simulink model "Feeder_1"  (Simulink 8.8)
settings: Solver=ode4  StartTime=0.0  StopTime=inf  FixedStep=Ts  RelTol=1e-3  EnableMultiTasking=on
PreLoadFcn:
  | Ts=125e-6;Core_Num = 0; np=1; nq=1; Vmin=.9;
PostLoadFcn:
  | Ts=125e-6;Core_Num = 0; np=1; nq=1; Vmin=.9;
InitFcn:
  | Ts=125e-6;Core_Num = 0; np=1; nq=1; Vmin=.9;
undefined symbols (not defined in the file or in its folder): another_event_name, DiscIntNeverNeededParam, I, j, Left, my_event_name, Right, type, V, X
libraries: powerlib x316, powerlib_meascontrol x227, simulink_extras x78, simulink x25, rtio_generic_c37_118 x22, ssn_lib x9, rtlab x6, powerlib_extras x3, artemis x1, rtio_opalrt_ml605ex1 x1, rtio_spectracom x1, rtio_generic_ethernet x1
(part 9 of 14)

== system Feeder_1/SM_NG/Single-Phase Dynamic Load41/model/Break  Alg. Loop1 ==
  In : Inport
  Complex to Real-Imag : ComplexToRealImag
  Real-Imag to Complex : RealImagToComplex
  imag : simulink_extras/Additional Linear/Transfer Fcn (with initial outputs)  N=[1]  D="[100e-6  1]"  Y0=imag(I1_init*exp(-j*Pha_V0*pi/180))  U0=imag(I1_init*exp(-j*Pha_V0*pi/180))
  real : simulink_extras/Additional Linear/Transfer Fcn (with initial outputs)  N=[1]  D="[100e-6  1]"  Y0=real(I1_init*exp(-j*Pha_V0*pi/180))  U0=real(I1_init*exp(-j*Pha_V0*pi/180))
  Out : Outport
  wires:
  Complex to Real-Imag/2 -> imag/1
  Complex to Real-Imag/1 -> real/1
  Real-Imag to Complex/1 -> Out/1
  In/1 -> Complex to Real-Imag/1
  imag/1 -> Real-Imag to Complex/2
  real/1 -> Real-Imag to Complex/1

== system Feeder_1/SM_NG/Single-Phase Dynamic Load41/model/PLL ==
  v (pu) : Inport
  freq (pu) : Inport  Port=2
  Gain : Gain  Gain=2*pi
  Gain1 : Gain  Gain=500
  Gain2 : Gain  Gain=freq
  IC : InitialCondition
  Integrator : Integrator
  Integrator1 : Integrator
  Product : Product  Inputs=**  RndMeth=Zero
  Sum1 : Sum  SaturateOnIntegerOverflow=on  InputSameDT=on  OutDataTypeStr=Inherit: Same as first input
  Trigonometric Function : Trigonometry  Operator=cos
  adaptive filter : Subsystem
  adaptive mean : Subsystem
  alpha (rad) : Outport
  wt : Outport  Port=2
  wires:
  freq (pu)/1 -> Gain2/1
  Gain2/1 -> adaptive filter/2(freq (Hz)), adaptive mean/2(freq (Hz)), Gain/1
  Trigonometric Function/1 -> Product/2
  adaptive mean/1(y) -> alpha (rad)/1
  Integrator1/1 -> Gain1/1
  Gain1/1 -> Sum1/1, adaptive mean/1(u)
  Sum1/1 -> Trigonometric Function/1
  Integrator/1 -> Sum1/2, wt/1
  Gain/1 -> Integrator/1
  adaptive filter/1(y) -> Integrator1/1
  Product/1 -> adaptive filter/1(u)
  v (pu)/1 -> IC/1
  IC/1 -> Product/1

== system Feeder_1/SM_NG/Single-Phase Dynamic Load41/model/Positive Sequence  current ==
  note: I1= (S/V1)'
  V1(pu) : Inport
  S_ext : Inport  Port=2
  Conj1 : Math  Operator=conj  SaturateOnIntegerOverflow=on
  Product : Product  Inputs=/*  SaturateOnIntegerOverflow=on  InputSameDT=on  OutDataTypeStr=Inherit: Same as first input
  pu>V : Gain  Gain=Vnom/sqrt(2)  SaturateOnIntegerOverflow=on  OutDataTypeStr=Inherit: Same as input  ParamDataTypeStr=Inherit: Same as input
  I1(A) : Outport
  wires:
  V1(pu)/1 -> pu>V/1
  Product/1 -> Conj1/1
  Conj1/1 -> I1(A)/1
  S_ext/1 -> Product/2
  pu>V/1 -> Product/1

== system Feeder_1/SM_NG/Single-Phase Dynamic Load42/model/Break  Alg. Loop1 ==
  In : Inport
  Complex to Real-Imag : ComplexToRealImag
  Real-Imag to Complex : RealImagToComplex
  imag : simulink_extras/Additional Linear/Transfer Fcn (with initial outputs)  N=[1]  D="[100e-6  1]"  Y0=imag(I1_init*exp(-j*Pha_V0*pi/180))  U0=imag(I1_init*exp(-j*Pha_V0*pi/180))
  real : simulink_extras/Additional Linear/Transfer Fcn (with initial outputs)  N=[1]  D="[100e-6  1]"  Y0=real(I1_init*exp(-j*Pha_V0*pi/180))  U0=real(I1_init*exp(-j*Pha_V0*pi/180))
  Out : Outport
  wires:
  Complex to Real-Imag/2 -> imag/1
  Complex to Real-Imag/1 -> real/1
  Real-Imag to Complex/1 -> Out/1
  In/1 -> Complex to Real-Imag/1
  imag/1 -> Real-Imag to Complex/2
  real/1 -> Real-Imag to Complex/1

== system Feeder_1/SM_NG/Single-Phase Dynamic Load42/model/PLL ==
  v (pu) : Inport
  freq (pu) : Inport  Port=2
  Gain : Gain  Gain=2*pi
  Gain1 : Gain  Gain=500
  Gain2 : Gain  Gain=freq
  IC : InitialCondition
  Integrator : Integrator
  Integrator1 : Integrator
  Product : Product  Inputs=**  RndMeth=Zero
  Sum1 : Sum  SaturateOnIntegerOverflow=on  InputSameDT=on  OutDataTypeStr=Inherit: Same as first input
  Trigonometric Function : Trigonometry  Operator=cos
  adaptive filter : Subsystem
  adaptive mean : Subsystem
  alpha (rad) : Outport
  wt : Outport  Port=2
  wires:
  freq (pu)/1 -> Gain2/1
  Gain2/1 -> adaptive filter/2(freq (Hz)), adaptive mean/2(freq (Hz)), Gain/1
  Trigonometric Function/1 -> Product/2
  adaptive mean/1(y) -> alpha (rad)/1
  Integrator1/1 -> Gain1/1
  Gain1/1 -> Sum1/1, adaptive mean/1(u)
  Sum1/1 -> Trigonometric Function/1
  Integrator/1 -> Sum1/2, wt/1
  Gain/1 -> Integrator/1
  adaptive filter/1(y) -> Integrator1/1
  Product/1 -> adaptive filter/1(u)
  v (pu)/1 -> IC/1
  IC/1 -> Product/1

== system Feeder_1/SM_NG/Single-Phase Dynamic Load42/model/Positive Sequence  current ==
  note: I1= (S/V1)'
  V1(pu) : Inport
  S_ext : Inport  Port=2
  Conj1 : Math  Operator=conj  SaturateOnIntegerOverflow=on
  Product : Product  Inputs=/*  SaturateOnIntegerOverflow=on  InputSameDT=on  OutDataTypeStr=Inherit: Same as first input
  pu>V : Gain  Gain=Vnom/sqrt(2)  SaturateOnIntegerOverflow=on  OutDataTypeStr=Inherit: Same as input  ParamDataTypeStr=Inherit: Same as input
  I1(A) : Outport
  wires:
  V1(pu)/1 -> pu>V/1
  Product/1 -> Conj1/1
  Conj1/1 -> I1(A)/1
  S_ext/1 -> Product/2
  pu>V/1 -> Product/1

== system Feeder_1/SM_NG/Single-Phase Dynamic Load43/model/Break  Alg. Loop1 ==
  In : Inport
  Complex to Real-Imag : ComplexToRealImag
  Real-Imag to Complex : RealImagToComplex
  imag : simulink_extras/Additional Linear/Transfer Fcn (with initial outputs)  N=[1]  D="[100e-6  1]"  Y0=imag(I1_init*exp(-j*Pha_V0*pi/180))  U0=imag(I1_init*exp(-j*Pha_V0*pi/180))
  real : simulink_extras/Additional Linear/Transfer Fcn (with initial outputs)  N=[1]  D="[100e-6  1]"  Y0=real(I1_init*exp(-j*Pha_V0*pi/180))  U0=real(I1_init*exp(-j*Pha_V0*pi/180))
  Out : Outport
  wires:
  Complex to Real-Imag/2 -> imag/1
  Complex to Real-Imag/1 -> real/1
  Real-Imag to Complex/1 -> Out/1
  In/1 -> Complex to Real-Imag/1
  imag/1 -> Real-Imag to Complex/2
  real/1 -> Real-Imag to Complex/1

== system Feeder_1/SM_NG/Single-Phase Dynamic Load43/model/PLL ==
  v (pu) : Inport
  freq (pu) : Inport  Port=2
  Gain : Gain  Gain=2*pi
  Gain1 : Gain  Gain=500
  Gain2 : Gain  Gain=freq
  IC : InitialCondition
  Integrator : Integrator
  Integrator1 : Integrator
  Product : Product  Inputs=**  RndMeth=Zero
  Sum1 : Sum  SaturateOnIntegerOverflow=on  InputSameDT=on  OutDataTypeStr=Inherit: Same as first input
  Trigonometric Function : Trigonometry  Operator=cos
  adaptive filter : Subsystem
  adaptive mean : Subsystem
  alpha (rad) : Outport
  wt : Outport  Port=2
  wires:
  freq (pu)/1 -> Gain2/1
  Gain2/1 -> adaptive filter/2(freq (Hz)), adaptive mean/2(freq (Hz)), Gain/1
  Trigonometric Function/1 -> Product/2
  adaptive mean/1(y) -> alpha (rad)/1
  Integrator1/1 -> Gain1/1
  Gain1/1 -> Sum1/1, adaptive mean/1(u)
  Sum1/1 -> Trigonometric Function/1
  Integrator/1 -> Sum1/2, wt/1
  Gain/1 -> Integrator/1
  adaptive filter/1(y) -> Integrator1/1
  Product/1 -> adaptive filter/1(u)
  v (pu)/1 -> IC/1
  IC/1 -> Product/1

== system Feeder_1/SM_NG/Single-Phase Dynamic Load43/model/Positive Sequence  current ==
  note: I1= (S/V1)'
  V1(pu) : Inport
  S_ext : Inport  Port=2
  Conj1 : Math  Operator=conj  SaturateOnIntegerOverflow=on
  Product : Product  Inputs=/*  SaturateOnIntegerOverflow=on  InputSameDT=on  OutDataTypeStr=Inherit: Same as first input
  pu>V : Gain  Gain=Vnom/sqrt(2)  SaturateOnIntegerOverflow=on  OutDataTypeStr=Inherit: Same as input  ParamDataTypeStr=Inherit: Same as input
  I1(A) : Outport
  wires:
  V1(pu)/1 -> pu>V/1
  Product/1 -> Conj1/1
  Conj1/1 -> I1(A)/1
  S_ext/1 -> Product/2
  pu>V/1 -> Product/1

== system Feeder_1/SM_NG/Single-Phase Dynamic Load44/model/Break  Alg. Loop1 ==
  In : Inport
  Complex to Real-Imag : ComplexToRealImag
  Real-Imag to Complex : RealImagToComplex
  imag : simulink_extras/Additional Linear/Transfer Fcn (with initial outputs)  N=[1]  D="[100e-6  1]"  Y0=imag(I1_init*exp(-j*Pha_V0*pi/180))  U0=imag(I1_init*exp(-j*Pha_V0*pi/180))
  real : simulink_extras/Additional Linear/Transfer Fcn (with initial outputs)  N=[1]  D="[100e-6  1]"  Y0=real(I1_init*exp(-j*Pha_V0*pi/180))  U0=real(I1_init*exp(-j*Pha_V0*pi/180))
  Out : Outport
  wires:
  Complex to Real-Imag/2 -> imag/1
  Complex to Real-Imag/1 -> real/1
  Real-Imag to Complex/1 -> Out/1
  In/1 -> Complex to Real-Imag/1
  imag/1 -> Real-Imag to Complex/2
  real/1 -> Real-Imag to Complex/1

== system Feeder_1/SM_NG/Single-Phase Dynamic Load44/model/PLL ==
  v (pu) : Inport
  freq (pu) : Inport  Port=2
  Gain : Gain  Gain=2*pi
  Gain1 : Gain  Gain=500
  Gain2 : Gain  Gain=freq
  IC : InitialCondition
  Integrator : Integrator
  Integrator1 : Integrator
  Product : Product  Inputs=**  RndMeth=Zero
  Sum1 : Sum  SaturateOnIntegerOverflow=on  InputSameDT=on  OutDataTypeStr=Inherit: Same as first input
  Trigonometric Function : Trigonometry  Operator=cos
  adaptive filter : Subsystem
  adaptive mean : Subsystem
  alpha (rad) : Outport
  wt : Outport  Port=2
  wires:
  freq (pu)/1 -> Gain2/1
  Gain2/1 -> adaptive filter/2(freq (Hz)), adaptive mean/2(freq (Hz)), Gain/1
  Trigonometric Function/1 -> Product/2
  adaptive mean/1(y) -> alpha (rad)/1
  Integrator1/1 -> Gain1/1
  Gain1/1 -> Sum1/1, adaptive mean/1(u)
  Sum1/1 -> Trigonometric Function/1
  Integrator/1 -> Sum1/2, wt/1
  Gain/1 -> Integrator/1
  adaptive filter/1(y) -> Integrator1/1
  Product/1 -> adaptive filter/1(u)
  v (pu)/1 -> IC/1
  IC/1 -> Product/1

== system Feeder_1/SM_NG/Single-Phase Dynamic Load44/model/Positive Sequence  current ==
  note: I1= (S/V1)'
  V1(pu) : Inport
  S_ext : Inport  Port=2
  Conj1 : Math  Operator=conj  SaturateOnIntegerOverflow=on
  Product : Product  Inputs=/*  SaturateOnIntegerOverflow=on  InputSameDT=on  OutDataTypeStr=Inherit: Same as first input
  pu>V : Gain  Gain=Vnom/sqrt(2)  SaturateOnIntegerOverflow=on  OutDataTypeStr=Inherit: Same as input  ParamDataTypeStr=Inherit: Same as input
  I1(A) : Outport
  wires:
  V1(pu)/1 -> pu>V/1
  Product/1 -> Conj1/1
  Conj1/1 -> I1(A)/1
  S_ext/1 -> Product/2
  pu>V/1 -> Product/1

== system Feeder_1/SM_NG/Single-Phase Dynamic Load45/model/Break  Alg. Loop1 ==
  In : Inport
  Complex to Real-Imag : ComplexToRealImag
  Real-Imag to Complex : RealImagToComplex
  imag : simulink_extras/Additional Linear/Transfer Fcn (with initial outputs)  N=[1]  D="[100e-6  1]"  Y0=imag(I1_init*exp(-j*Pha_V0*pi/180))  U0=imag(I1_init*exp(-j*Pha_V0*pi/180))
  real : simulink_extras/Additional Linear/Transfer Fcn (with initial outputs)  N=[1]  D="[100e-6  1]"  Y0=real(I1_init*exp(-j*Pha_V0*pi/180))  U0=real(I1_init*exp(-j*Pha_V0*pi/180))
  Out : Outport
  wires:
  Complex to Real-Imag/2 -> imag/1
  Complex to Real-Imag/1 -> real/1
  Real-Imag to Complex/1 -> Out/1
  In/1 -> Complex to Real-Imag/1
  imag/1 -> Real-Imag to Complex/2
  real/1 -> Real-Imag to Complex/1

== system Feeder_1/SM_NG/Single-Phase Dynamic Load45/model/PLL ==
  v (pu) : Inport
  freq (pu) : Inport  Port=2
  Gain : Gain  Gain=2*pi
  Gain1 : Gain  Gain=500
  Gain2 : Gain  Gain=freq
  IC : InitialCondition
  Integrator : Integrator
  Integrator1 : Integrator
  Product : Product  Inputs=**  RndMeth=Zero
  Sum1 : Sum  SaturateOnIntegerOverflow=on  InputSameDT=on  OutDataTypeStr=Inherit: Same as first input
  Trigonometric Function : Trigonometry  Operator=cos
  adaptive filter : Subsystem
  adaptive mean : Subsystem
  alpha (rad) : Outport
  wt : Outport  Port=2
  wires:
  freq (pu)/1 -> Gain2/1
  Gain2/1 -> adaptive filter/2(freq (Hz)), adaptive mean/2(freq (Hz)), Gain/1
  Trigonometric Function/1 -> Product/2
  adaptive mean/1(y) -> alpha (rad)/1
  Integrator1/1 -> Gain1/1
  Gain1/1 -> Sum1/1, adaptive mean/1(u)
  Sum1/1 -> Trigonometric Function/1
  Integrator/1 -> Sum1/2, wt/1
  Gain/1 -> Integrator/1
  adaptive filter/1(y) -> Integrator1/1
  Product/1 -> adaptive filter/1(u)
  v (pu)/1 -> IC/1
  IC/1 -> Product/1

== system Feeder_1/SM_NG/Single-Phase Dynamic Load45/model/Positive Sequence  current ==
  note: I1= (S/V1)'
  V1(pu) : Inport
  S_ext : Inport  Port=2
  Conj1 : Math  Operator=conj  SaturateOnIntegerOverflow=on
  Product : Product  Inputs=/*  SaturateOnIntegerOverflow=on  InputSameDT=on  OutDataTypeStr=Inherit: Same as first input
  pu>V : Gain  Gain=Vnom/sqrt(2)  SaturateOnIntegerOverflow=on  OutDataTypeStr=Inherit: Same as input  ParamDataTypeStr=Inherit: Same as input
  I1(A) : Outport
  wires:
  V1(pu)/1 -> pu>V/1
  Product/1 -> Conj1/1
  Conj1/1 -> I1(A)/1
  S_ext/1 -> Product/2
  pu>V/1 -> Product/1

== system Feeder_1/SM_NG/Single-Phase Dynamic Load46/model/Break  Alg. Loop1 ==
  In : Inport
  Complex to Real-Imag : ComplexToRealImag
  Real-Imag to Complex : RealImagToComplex
  imag : simulink_extras/Additional Linear/Transfer Fcn (with initial outputs)  N=[1]  D="[100e-6  1]"  Y0=imag(I1_init*exp(-j*Pha_V0*pi/180))  U0=imag(I1_init*exp(-j*Pha_V0*pi/180))
  real : simulink_extras/Additional Linear/Transfer Fcn (with initial outputs)  N=[1]  D="[100e-6  1]"  Y0=real(I1_init*exp(-j*Pha_V0*pi/180))  U0=real(I1_init*exp(-j*Pha_V0*pi/180))
  Out : Outport
  wires:
  Complex to Real-Imag/2 -> imag/1
  Complex to Real-Imag/1 -> real/1
  Real-Imag to Complex/1 -> Out/1
  In/1 -> Complex to Real-Imag/1
  imag/1 -> Real-Imag to Complex/2
  real/1 -> Real-Imag to Complex/1

== system Feeder_1/SM_NG/Single-Phase Dynamic Load46/model/PLL ==
  v (pu) : Inport
  freq (pu) : Inport  Port=2
  Gain : Gain  Gain=2*pi
  Gain1 : Gain  Gain=500
  Gain2 : Gain  Gain=freq
  IC : InitialCondition
  Integrator : Integrator
  Integrator1 : Integrator
  Product : Product  Inputs=**  RndMeth=Zero
  Sum1 : Sum  SaturateOnIntegerOverflow=on  InputSameDT=on  OutDataTypeStr=Inherit: Same as first input
  Trigonometric Function : Trigonometry  Operator=cos
  adaptive filter : Subsystem
  adaptive mean : Subsystem
  alpha (rad) : Outport
  wt : Outport  Port=2
  wires:
  freq (pu)/1 -> Gain2/1
  Gain2/1 -> adaptive filter/2(freq (Hz)), adaptive mean/2(freq (Hz)), Gain/1
  Trigonometric Function/1 -> Product/2
  adaptive mean/1(y) -> alpha (rad)/1
  Integrator1/1 -> Gain1/1
  Gain1/1 -> Sum1/1, adaptive mean/1(u)
  Sum1/1 -> Trigonometric Function/1
  Integrator/1 -> Sum1/2, wt/1
  Gain/1 -> Integrator/1
  adaptive filter/1(y) -> Integrator1/1
  Product/1 -> adaptive filter/1(u)
  v (pu)/1 -> IC/1
  IC/1 -> Product/1

== system Feeder_1/SM_NG/Single-Phase Dynamic Load46/model/Positive Sequence  current ==
  note: I1= (S/V1)'
  V1(pu) : Inport
  S_ext : Inport  Port=2
  Conj1 : Math  Operator=conj  SaturateOnIntegerOverflow=on
  Product : Product  Inputs=/*  SaturateOnIntegerOverflow=on  InputSameDT=on  OutDataTypeStr=Inherit: Same as first input
  pu>V : Gain  Gain=Vnom/sqrt(2)  SaturateOnIntegerOverflow=on  OutDataTypeStr=Inherit: Same as input  ParamDataTypeStr=Inherit: Same as input
  I1(A) : Outport
  wires:
  V1(pu)/1 -> pu>V/1
  Product/1 -> Conj1/1
  Conj1/1 -> I1(A)/1
  S_ext/1 -> Product/2
  pu>V/1 -> Product/1

== system Feeder_1/SM_NG/Single-Phase Dynamic Load47/model/Break  Alg. Loop1 ==
  In : Inport
  Complex to Real-Imag : ComplexToRealImag
  Real-Imag to Complex : RealImagToComplex
  imag : simulink_extras/Additional Linear/Transfer Fcn (with initial outputs)  N=[1]  D="[100e-6  1]"  Y0=imag(I1_init*exp(-j*Pha_V0*pi/180))  U0=imag(I1_init*exp(-j*Pha_V0*pi/180))
  real : simulink_extras/Additional Linear/Transfer Fcn (with initial outputs)  N=[1]  D="[100e-6  1]"  Y0=real(I1_init*exp(-j*Pha_V0*pi/180))  U0=real(I1_init*exp(-j*Pha_V0*pi/180))
  Out : Outport
  wires:
  Complex to Real-Imag/2 -> imag/1
  Complex to Real-Imag/1 -> real/1
  Real-Imag to Complex/1 -> Out/1
  In/1 -> Complex to Real-Imag/1
  imag/1 -> Real-Imag to Complex/2
  real/1 -> Real-Imag to Complex/1

== system Feeder_1/SM_NG/Single-Phase Dynamic Load47/model/PLL ==
  v (pu) : Inport
  freq (pu) : Inport  Port=2
  Gain : Gain  Gain=2*pi
  Gain1 : Gain  Gain=500
  Gain2 : Gain  Gain=freq
  IC : InitialCondition
  Integrator : Integrator
  Integrator1 : Integrator
  Product : Product  Inputs=**  RndMeth=Zero
  Sum1 : Sum  SaturateOnIntegerOverflow=on  InputSameDT=on  OutDataTypeStr=Inherit: Same as first input
  Trigonometric Function : Trigonometry  Operator=cos
  adaptive filter : Subsystem
  adaptive mean : Subsystem
  alpha (rad) : Outport
  wt : Outport  Port=2
  wires:
  freq (pu)/1 -> Gain2/1
  Gain2/1 -> adaptive filter/2(freq (Hz)), adaptive mean/2(freq (Hz)), Gain/1
  Trigonometric Function/1 -> Product/2
  adaptive mean/1(y) -> alpha (rad)/1
  Integrator1/1 -> Gain1/1
  Gain1/1 -> Sum1/1, adaptive mean/1(u)
  Sum1/1 -> Trigonometric Function/1
  Integrator/1 -> Sum1/2, wt/1
  Gain/1 -> Integrator/1
  adaptive filter/1(y) -> Integrator1/1
  Product/1 -> adaptive filter/1(u)
  v (pu)/1 -> IC/1
  IC/1 -> Product/1

== system Feeder_1/SM_NG/Single-Phase Dynamic Load47/model/Positive Sequence  current ==
  note: I1= (S/V1)'
  V1(pu) : Inport
  S_ext : Inport  Port=2
  Conj1 : Math  Operator=conj  SaturateOnIntegerOverflow=on
  Product : Product  Inputs=/*  SaturateOnIntegerOverflow=on  InputSameDT=on  OutDataTypeStr=Inherit: Same as first input
  pu>V : Gain  Gain=Vnom/sqrt(2)  SaturateOnIntegerOverflow=on  OutDataTypeStr=Inherit: Same as input  ParamDataTypeStr=Inherit: Same as input
  I1(A) : Outport
  wires:
  V1(pu)/1 -> pu>V/1
  Product/1 -> Conj1/1
  Conj1/1 -> I1(A)/1
  S_ext/1 -> Product/2
  pu>V/1 -> Product/1

== system Feeder_1/SM_NG/Single-Phase Dynamic Load48/model/Break  Alg. Loop1 ==
  In : Inport
  Complex to Real-Imag : ComplexToRealImag
  Real-Imag to Complex : RealImagToComplex
  imag : simulink_extras/Additional Linear/Transfer Fcn (with initial outputs)  N=[1]  D="[100e-6  1]"  Y0=imag(I1_init*exp(-j*Pha_V0*pi/180))  U0=imag(I1_init*exp(-j*Pha_V0*pi/180))
  real : simulink_extras/Additional Linear/Transfer Fcn (with initial outputs)  N=[1]  D="[100e-6  1]"  Y0=real(I1_init*exp(-j*Pha_V0*pi/180))  U0=real(I1_init*exp(-j*Pha_V0*pi/180))
  Out : Outport
  wires:
  Complex to Real-Imag/2 -> imag/1
  Complex to Real-Imag/1 -> real/1
  Real-Imag to Complex/1 -> Out/1
  In/1 -> Complex to Real-Imag/1
  imag/1 -> Real-Imag to Complex/2
  real/1 -> Real-Imag to Complex/1

== system Feeder_1/SM_NG/Single-Phase Dynamic Load48/model/PLL ==
  v (pu) : Inport
  freq (pu) : Inport  Port=2
  Gain : Gain  Gain=2*pi
  Gain1 : Gain  Gain=500
  Gain2 : Gain  Gain=freq
  IC : InitialCondition
  Integrator : Integrator
  Integrator1 : Integrator
  Product : Product  Inputs=**  RndMeth=Zero
  Sum1 : Sum  SaturateOnIntegerOverflow=on  InputSameDT=on  OutDataTypeStr=Inherit: Same as first input
  Trigonometric Function : Trigonometry  Operator=cos
  adaptive filter : Subsystem
  adaptive mean : Subsystem
  alpha (rad) : Outport
  wt : Outport  Port=2
  wires:
  freq (pu)/1 -> Gain2/1
  Gain2/1 -> adaptive filter/2(freq (Hz)), adaptive mean/2(freq (Hz)), Gain/1
  Trigonometric Function/1 -> Product/2
  adaptive mean/1(y) -> alpha (rad)/1
  Integrator1/1 -> Gain1/1
  Gain1/1 -> Sum1/1, adaptive mean/1(u)
  Sum1/1 -> Trigonometric Function/1
  Integrator/1 -> Sum1/2, wt/1
  Gain/1 -> Integrator/1
  adaptive filter/1(y) -> Integrator1/1
  Product/1 -> adaptive filter/1(u)
  v (pu)/1 -> IC/1
  IC/1 -> Product/1

== system Feeder_1/SM_NG/Single-Phase Dynamic Load48/model/Positive Sequence  current ==
  note: I1= (S/V1)'
  V1(pu) : Inport
  S_ext : Inport  Port=2
  Conj1 : Math  Operator=conj  SaturateOnIntegerOverflow=on
  Product : Product  Inputs=/*  SaturateOnIntegerOverflow=on  InputSameDT=on  OutDataTypeStr=Inherit: Same as first input
  pu>V : Gain  Gain=Vnom/sqrt(2)  SaturateOnIntegerOverflow=on  OutDataTypeStr=Inherit: Same as input  ParamDataTypeStr=Inherit: Same as input
  I1(A) : Outport
  wires:
  V1(pu)/1 -> pu>V/1
  Product/1 -> Conj1/1
  Conj1/1 -> I1(A)/1
  S_ext/1 -> Product/2
  pu>V/1 -> Product/1

== system Feeder_1/SM_NG/Single-Phase Dynamic Load49/model/Break  Alg. Loop1 ==
  In : Inport
  Complex to Real-Imag : ComplexToRealImag
  Real-Imag to Complex : RealImagToComplex
  imag : simulink_extras/Additional Linear/Transfer Fcn (with initial outputs)  N=[1]  D="[100e-6  1]"  Y0=imag(I1_init*exp(-j*Pha_V0*pi/180))  U0=imag(I1_init*exp(-j*Pha_V0*pi/180))
  real : simulink_extras/Additional Linear/Transfer Fcn (with initial outputs)  N=[1]  D="[100e-6  1]"  Y0=real(I1_init*exp(-j*Pha_V0*pi/180))  U0=real(I1_init*exp(-j*Pha_V0*pi/180))
  Out : Outport
  wires:
  Complex to Real-Imag/2 -> imag/1
  Complex to Real-Imag/1 -> real/1
  Real-Imag to Complex/1 -> Out/1
  In/1 -> Complex to Real-Imag/1
  imag/1 -> Real-Imag to Complex/2
  real/1 -> Real-Imag to Complex/1

== system Feeder_1/SM_NG/Single-Phase Dynamic Load49/model/PLL ==
  v (pu) : Inport
  freq (pu) : Inport  Port=2
  Gain : Gain  Gain=2*pi
  Gain1 : Gain  Gain=500
  Gain2 : Gain  Gain=freq
  IC : InitialCondition
  Integrator : Integrator
  Integrator1 : Integrator
  Product : Product  Inputs=**  RndMeth=Zero
  Sum1 : Sum  SaturateOnIntegerOverflow=on  InputSameDT=on  OutDataTypeStr=Inherit: Same as first input
  Trigonometric Function : Trigonometry  Operator=cos
  adaptive filter : Subsystem
  adaptive mean : Subsystem
  alpha (rad) : Outport
  wt : Outport  Port=2
  wires:
  freq (pu)/1 -> Gain2/1
  Gain2/1 -> adaptive filter/2(freq (Hz)), adaptive mean/2(freq (Hz)), Gain/1
  Trigonometric Function/1 -> Product/2
  adaptive mean/1(y) -> alpha (rad)/1
  Integrator1/1 -> Gain1/1
  Gain1/1 -> Sum1/1, adaptive mean/1(u)
  Sum1/1 -> Trigonometric Function/1
  Integrator/1 -> Sum1/2, wt/1
  Gain/1 -> Integrator/1
  adaptive filter/1(y) -> Integrator1/1
  Product/1 -> adaptive filter/1(u)
  v (pu)/1 -> IC/1
  IC/1 -> Product/1

== system Feeder_1/SM_NG/Single-Phase Dynamic Load49/model/Positive Sequence  current ==
  note: I1= (S/V1)'
  V1(pu) : Inport
  S_ext : Inport  Port=2
  Conj1 : Math  Operator=conj  SaturateOnIntegerOverflow=on
  Product : Product  Inputs=/*  SaturateOnIntegerOverflow=on  InputSameDT=on  OutDataTypeStr=Inherit: Same as first input
  pu>V : Gain  Gain=Vnom/sqrt(2)  SaturateOnIntegerOverflow=on  OutDataTypeStr=Inherit: Same as input  ParamDataTypeStr=Inherit: Same as input
  I1(A) : Outport
  wires:
  V1(pu)/1 -> pu>V/1
  Product/1 -> Conj1/1
  Conj1/1 -> I1(A)/1
  S_ext/1 -> Product/2
  pu>V/1 -> Product/1

== system Feeder_1/SM_NG/Single-Phase Dynamic Load50/model/Break  Alg. Loop1 ==
  In : Inport
  Complex to Real-Imag : ComplexToRealImag
  Real-Imag to Complex : RealImagToComplex
  imag : simulink_extras/Additional Linear/Transfer Fcn (with initial outputs)  N=[1]  D="[100e-6  1]"  Y0=imag(I1_init*exp(-j*Pha_V0*pi/180))  U0=imag(I1_init*exp(-j*Pha_V0*pi/180))
  real : simulink_extras/Additional Linear/Transfer Fcn (with initial outputs)  N=[1]  D="[100e-6  1]"  Y0=real(I1_init*exp(-j*Pha_V0*pi/180))  U0=real(I1_init*exp(-j*Pha_V0*pi/180))
  Out : Outport
  wires:
  Complex to Real-Imag/2 -> imag/1
  Complex to Real-Imag/1 -> real/1
  Real-Imag to Complex/1 -> Out/1
  In/1 -> Complex to Real-Imag/1
  imag/1 -> Real-Imag to Complex/2
  real/1 -> Real-Imag to Complex/1

== system Feeder_1/SM_NG/Single-Phase Dynamic Load50/model/PLL ==
  v (pu) : Inport
  freq (pu) : Inport  Port=2
  Gain : Gain  Gain=2*pi
  Gain1 : Gain  Gain=500
  Gain2 : Gain  Gain=freq
  IC : InitialCondition
  Integrator : Integrator
  Integrator1 : Integrator
  Product : Product  Inputs=**  RndMeth=Zero
  Sum1 : Sum  SaturateOnIntegerOverflow=on  InputSameDT=on  OutDataTypeStr=Inherit: Same as first input
  Trigonometric Function : Trigonometry  Operator=cos
  adaptive filter : Subsystem
  adaptive mean : Subsystem
  alpha (rad) : Outport
  wt : Outport  Port=2
  wires:
  freq (pu)/1 -> Gain2/1
  Gain2/1 -> adaptive filter/2(freq (Hz)), adaptive mean/2(freq (Hz)), Gain/1
  Trigonometric Function/1 -> Product/2
  adaptive mean/1(y) -> alpha (rad)/1
  Integrator1/1 -> Gain1/1
  Gain1/1 -> Sum1/1, adaptive mean/1(u)
  Sum1/1 -> Trigonometric Function/1
  Integrator/1 -> Sum1/2, wt/1
  Gain/1 -> Integrator/1
  adaptive filter/1(y) -> Integrator1/1
  Product/1 -> adaptive filter/1(u)
  v (pu)/1 -> IC/1
  IC/1 -> Product/1

== system Feeder_1/SM_NG/Single-Phase Dynamic Load50/model/Positive Sequence  current ==
  note: I1= (S/V1)'
  V1(pu) : Inport
  S_ext : Inport  Port=2
  Conj1 : Math  Operator=conj  SaturateOnIntegerOverflow=on
  Product : Product  Inputs=/*  SaturateOnIntegerOverflow=on  InputSameDT=on  OutDataTypeStr=Inherit: Same as first input
  pu>V : Gain  Gain=Vnom/sqrt(2)  SaturateOnIntegerOverflow=on  OutDataTypeStr=Inherit: Same as input  ParamDataTypeStr=Inherit: Same as input
  I1(A) : Outport
  wires:
  V1(pu)/1 -> pu>V/1
  Product/1 -> Conj1/1
  Conj1/1 -> I1(A)/1
  S_ext/1 -> Product/2
  pu>V/1 -> Product/1

== system Feeder_1/SM_NG/Single-Phase Dynamic Load51/model/Break  Alg. Loop1 ==
  In : Inport
  Complex to Real-Imag : ComplexToRealImag
  Real-Imag to Complex : RealImagToComplex
  imag : simulink_extras/Additional Linear/Transfer Fcn (with initial outputs)  N=[1]  D="[100e-6  1]"  Y0=imag(I1_init*exp(-j*Pha_V0*pi/180))  U0=imag(I1_init*exp(-j*Pha_V0*pi/180))
  real : simulink_extras/Additional Linear/Transfer Fcn (with initial outputs)  N=[1]  D="[100e-6  1]"  Y0=real(I1_init*exp(-j*Pha_V0*pi/180))  U0=real(I1_init*exp(-j*Pha_V0*pi/180))
  Out : Outport
  wires:
  Complex to Real-Imag/2 -> imag/1
  Complex to Real-Imag/1 -> real/1
  Real-Imag to Complex/1 -> Out/1
  In/1 -> Complex to Real-Imag/1
  imag/1 -> Real-Imag to Complex/2
  real/1 -> Real-Imag to Complex/1

== system Feeder_1/SM_NG/Single-Phase Dynamic Load51/model/PLL ==
  v (pu) : Inport
  freq (pu) : Inport  Port=2
  Gain : Gain  Gain=2*pi
  Gain1 : Gain  Gain=500
  Gain2 : Gain  Gain=freq
  IC : InitialCondition
  Integrator : Integrator
  Integrator1 : Integrator
  Product : Product  Inputs=**  RndMeth=Zero
  Sum1 : Sum  SaturateOnIntegerOverflow=on  InputSameDT=on  OutDataTypeStr=Inherit: Same as first input
  Trigonometric Function : Trigonometry  Operator=cos
  adaptive filter : Subsystem
  adaptive mean : Subsystem
  alpha (rad) : Outport
  wt : Outport  Port=2
  wires:
  freq (pu)/1 -> Gain2/1
  Gain2/1 -> adaptive filter/2(freq (Hz)), adaptive mean/2(freq (Hz)), Gain/1
  Trigonometric Function/1 -> Product/2
  adaptive mean/1(y) -> alpha (rad)/1
  Integrator1/1 -> Gain1/1
  Gain1/1 -> Sum1/1, adaptive mean/1(u)
  Sum1/1 -> Trigonometric Function/1
  Integrator/1 -> Sum1/2, wt/1
  Gain/1 -> Integrator/1
  adaptive filter/1(y) -> Integrator1/1
  Product/1 -> adaptive filter/1(u)
  v (pu)/1 -> IC/1
  IC/1 -> Product/1

== system Feeder_1/SM_NG/Single-Phase Dynamic Load51/model/Positive Sequence  current ==
  note: I1= (S/V1)'
  V1(pu) : Inport
  S_ext : Inport  Port=2
  Conj1 : Math  Operator=conj  SaturateOnIntegerOverflow=on
  Product : Product  Inputs=/*  SaturateOnIntegerOverflow=on  InputSameDT=on  OutDataTypeStr=Inherit: Same as first input
  pu>V : Gain  Gain=Vnom/sqrt(2)  SaturateOnIntegerOverflow=on  OutDataTypeStr=Inherit: Same as input  ParamDataTypeStr=Inherit: Same as input
  I1(A) : Outport
  wires:
  V1(pu)/1 -> pu>V/1
  Product/1 -> Conj1/1
  Conj1/1 -> I1(A)/1
  S_ext/1 -> Product/2
  pu>V/1 -> Product/1

== system Feeder_1/SM_NG/Single-Phase Dynamic Load52/model/Break  Alg. Loop1 ==
  In : Inport
  Complex to Real-Imag : ComplexToRealImag
  Real-Imag to Complex : RealImagToComplex
  imag : simulink_extras/Additional Linear/Transfer Fcn (with initial outputs)  N=[1]  D="[100e-6  1]"  Y0=imag(I1_init*exp(-j*Pha_V0*pi/180))  U0=imag(I1_init*exp(-j*Pha_V0*pi/180))
  real : simulink_extras/Additional Linear/Transfer Fcn (with initial outputs)  N=[1]  D="[100e-6  1]"  Y0=real(I1_init*exp(-j*Pha_V0*pi/180))  U0=real(I1_init*exp(-j*Pha_V0*pi/180))
  Out : Outport
  wires:
  Complex to Real-Imag/2 -> imag/1
  Complex to Real-Imag/1 -> real/1
  Real-Imag to Complex/1 -> Out/1
  In/1 -> Complex to Real-Imag/1
  imag/1 -> Real-Imag to Complex/2
  real/1 -> Real-Imag to Complex/1

== system Feeder_1/SM_NG/Single-Phase Dynamic Load52/model/PLL ==
  v (pu) : Inport
  freq (pu) : Inport  Port=2
  Gain : Gain  Gain=2*pi
  Gain1 : Gain  Gain=500
  Gain2 : Gain  Gain=freq
  IC : InitialCondition
  Integrator : Integrator
  Integrator1 : Integrator
  Product : Product  Inputs=**  RndMeth=Zero
  Sum1 : Sum  SaturateOnIntegerOverflow=on  InputSameDT=on  OutDataTypeStr=Inherit: Same as first input
  Trigonometric Function : Trigonometry  Operator=cos
  adaptive filter : Subsystem
  adaptive mean : Subsystem
  alpha (rad) : Outport
  wt : Outport  Port=2
  wires:
  freq (pu)/1 -> Gain2/1
  Gain2/1 -> adaptive filter/2(freq (Hz)), adaptive mean/2(freq (Hz)), Gain/1
  Trigonometric Function/1 -> Product/2
  adaptive mean/1(y) -> alpha (rad)/1
  Integrator1/1 -> Gain1/1
  Gain1/1 -> Sum1/1, adaptive mean/1(u)
  Sum1/1 -> Trigonometric Function/1
  Integrator/1 -> Sum1/2, wt/1
  Gain/1 -> Integrator/1
  adaptive filter/1(y) -> Integrator1/1
  Product/1 -> adaptive filter/1(u)
  v (pu)/1 -> IC/1
  IC/1 -> Product/1

== system Feeder_1/SM_NG/Single-Phase Dynamic Load52/model/Positive Sequence  current ==
  note: I1= (S/V1)'
  V1(pu) : Inport
  S_ext : Inport  Port=2
  Conj1 : Math  Operator=conj  SaturateOnIntegerOverflow=on
  Product : Product  Inputs=/*  SaturateOnIntegerOverflow=on  InputSameDT=on  OutDataTypeStr=Inherit: Same as first input
  pu>V : Gain  Gain=Vnom/sqrt(2)  SaturateOnIntegerOverflow=on  OutDataTypeStr=Inherit: Same as input  ParamDataTypeStr=Inherit: Same as input
  I1(A) : Outport
  wires:
  V1(pu)/1 -> pu>V/1
  Product/1 -> Conj1/1
  Conj1/1 -> I1(A)/1
  S_ext/1 -> Product/2
  pu>V/1 -> Product/1

== system Feeder_1/SM_NG/Single-Phase Dynamic Load53/model/Break  Alg. Loop1 ==
  In : Inport
  Complex to Real-Imag : ComplexToRealImag
  Real-Imag to Complex : RealImagToComplex
  imag : simulink_extras/Additional Linear/Transfer Fcn (with initial outputs)  N=[1]  D="[100e-6  1]"  Y0=imag(I1_init*exp(-j*Pha_V0*pi/180))  U0=imag(I1_init*exp(-j*Pha_V0*pi/180))
  real : simulink_extras/Additional Linear/Transfer Fcn (with initial outputs)  N=[1]  D="[100e-6  1]"  Y0=real(I1_init*exp(-j*Pha_V0*pi/180))  U0=real(I1_init*exp(-j*Pha_V0*pi/180))
  Out : Outport
  wires:
  Complex to Real-Imag/2 -> imag/1
  Complex to Real-Imag/1 -> real/1
  Real-Imag to Complex/1 -> Out/1
  In/1 -> Complex to Real-Imag/1
  imag/1 -> Real-Imag to Complex/2
  real/1 -> Real-Imag to Complex/1

== system Feeder_1/SM_NG/Single-Phase Dynamic Load53/model/PLL ==
  v (pu) : Inport
  freq (pu) : Inport  Port=2
  Gain : Gain  Gain=2*pi
  Gain1 : Gain  Gain=500
  Gain2 : Gain  Gain=freq
  IC : InitialCondition
  Integrator : Integrator
  Integrator1 : Integrator
  Product : Product  Inputs=**  RndMeth=Zero
  Sum1 : Sum  SaturateOnIntegerOverflow=on  InputSameDT=on  OutDataTypeStr=Inherit: Same as first input
  Trigonometric Function : Trigonometry  Operator=cos
  adaptive filter : Subsystem
  adaptive mean : Subsystem
  alpha (rad) : Outport
  wt : Outport  Port=2
  wires:
  freq (pu)/1 -> Gain2/1
  Gain2/1 -> adaptive filter/2(freq (Hz)), adaptive mean/2(freq (Hz)), Gain/1
  Trigonometric Function/1 -> Product/2
  adaptive mean/1(y) -> alpha (rad)/1
  Integrator1/1 -> Gain1/1
  Gain1/1 -> Sum1/1, adaptive mean/1(u)
  Sum1/1 -> Trigonometric Function/1
  Integrator/1 -> Sum1/2, wt/1
  Gain/1 -> Integrator/1
  adaptive filter/1(y) -> Integrator1/1
  Product/1 -> adaptive filter/1(u)
  v (pu)/1 -> IC/1
  IC/1 -> Product/1

== system Feeder_1/SM_NG/Single-Phase Dynamic Load53/model/Positive Sequence  current ==
  note: I1= (S/V1)'
  V1(pu) : Inport
  S_ext : Inport  Port=2
  Conj1 : Math  Operator=conj  SaturateOnIntegerOverflow=on
  Product : Product  Inputs=/*  SaturateOnIntegerOverflow=on  InputSameDT=on  OutDataTypeStr=Inherit: Same as first input
  pu>V : Gain  Gain=Vnom/sqrt(2)  SaturateOnIntegerOverflow=on  OutDataTypeStr=Inherit: Same as input  ParamDataTypeStr=Inherit: Same as input
  I1(A) : Outport
  wires:
  V1(pu)/1 -> pu>V/1
  Product/1 -> Conj1/1
  Conj1/1 -> I1(A)/1
  S_ext/1 -> Product/2
  pu>V/1 -> Product/1

== system Feeder_1/SM_NG/Single-Phase Dynamic Load54/model/Break  Alg. Loop1 ==
  In : Inport
  Complex to Real-Imag : ComplexToRealImag
  Real-Imag to Complex : RealImagToComplex
  imag : simulink_extras/Additional Linear/Transfer Fcn (with initial outputs)  N=[1]  D="[100e-6  1]"  Y0=imag(I1_init*exp(-j*Pha_V0*pi/180))  U0=imag(I1_init*exp(-j*Pha_V0*pi/180))
  real : simulink_extras/Additional Linear/Transfer Fcn (with initial outputs)  N=[1]  D="[100e-6  1]"  Y0=real(I1_init*exp(-j*Pha_V0*pi/180))  U0=real(I1_init*exp(-j*Pha_V0*pi/180))
  Out : Outport
  wires:
  Complex to Real-Imag/2 -> imag/1
  Complex to Real-Imag/1 -> real/1
  Real-Imag to Complex/1 -> Out/1
  In/1 -> Complex to Real-Imag/1
  imag/1 -> Real-Imag to Complex/2
  real/1 -> Real-Imag to Complex/1

== system Feeder_1/SM_NG/Single-Phase Dynamic Load54/model/PLL ==
  v (pu) : Inport
  freq (pu) : Inport  Port=2
  Gain : Gain  Gain=2*pi
  Gain1 : Gain  Gain=500
  Gain2 : Gain  Gain=freq
  IC : InitialCondition
  Integrator : Integrator
  Integrator1 : Integrator
  Product : Product  Inputs=**  RndMeth=Zero
  Sum1 : Sum  SaturateOnIntegerOverflow=on  InputSameDT=on  OutDataTypeStr=Inherit: Same as first input
  Trigonometric Function : Trigonometry  Operator=cos
  adaptive filter : Subsystem
  adaptive mean : Subsystem
  alpha (rad) : Outport
  wt : Outport  Port=2
  wires:
  freq (pu)/1 -> Gain2/1
  Gain2/1 -> adaptive filter/2(freq (Hz)), adaptive mean/2(freq (Hz)), Gain/1
  Trigonometric Function/1 -> Product/2
  adaptive mean/1(y) -> alpha (rad)/1
  Integrator1/1 -> Gain1/1
  Gain1/1 -> Sum1/1, adaptive mean/1(u)
  Sum1/1 -> Trigonometric Function/1
  Integrator/1 -> Sum1/2, wt/1
  Gain/1 -> Integrator/1
  adaptive filter/1(y) -> Integrator1/1
  Product/1 -> adaptive filter/1(u)
  v (pu)/1 -> IC/1
  IC/1 -> Product/1

== system Feeder_1/SM_NG/Single-Phase Dynamic Load54/model/Positive Sequence  current ==
  note: I1= (S/V1)'
  V1(pu) : Inport
  S_ext : Inport  Port=2
  Conj1 : Math  Operator=conj  SaturateOnIntegerOverflow=on
  Product : Product  Inputs=/*  SaturateOnIntegerOverflow=on  InputSameDT=on  OutDataTypeStr=Inherit: Same as first input
  pu>V : Gain  Gain=Vnom/sqrt(2)  SaturateOnIntegerOverflow=on  OutDataTypeStr=Inherit: Same as input  ParamDataTypeStr=Inherit: Same as input
  I1(A) : Outport
  wires:
  V1(pu)/1 -> pu>V/1
  Product/1 -> Conj1/1
  Conj1/1 -> I1(A)/1
  S_ext/1 -> Product/2
  pu>V/1 -> Product/1

== system Feeder_1/SM_NG/Single-Phase Dynamic Load55/model/Break  Alg. Loop1 ==
  In : Inport
  Complex to Real-Imag : ComplexToRealImag
  Real-Imag to Complex : RealImagToComplex
  imag : simulink_extras/Additional Linear/Transfer Fcn (with initial outputs)  N=[1]  D="[100e-6  1]"  Y0=imag(I1_init*exp(-j*Pha_V0*pi/180))  U0=imag(I1_init*exp(-j*Pha_V0*pi/180))
  real : simulink_extras/Additional Linear/Transfer Fcn (with initial outputs)  N=[1]  D="[100e-6  1]"  Y0=real(I1_init*exp(-j*Pha_V0*pi/180))  U0=real(I1_init*exp(-j*Pha_V0*pi/180))
  Out : Outport
  wires:
  Complex to Real-Imag/2 -> imag/1
  Complex to Real-Imag/1 -> real/1
  Real-Imag to Complex/1 -> Out/1
  In/1 -> Complex to Real-Imag/1
  imag/1 -> Real-Imag to Complex/2
  real/1 -> Real-Imag to Complex/1

== system Feeder_1/SM_NG/Single-Phase Dynamic Load55/model/PLL ==
  v (pu) : Inport
  freq (pu) : Inport  Port=2
  Gain : Gain  Gain=2*pi
  Gain1 : Gain  Gain=500
  Gain2 : Gain  Gain=freq
  IC : InitialCondition
  Integrator : Integrator
  Integrator1 : Integrator
  Product : Product  Inputs=**  RndMeth=Zero
  Sum1 : Sum  SaturateOnIntegerOverflow=on  InputSameDT=on  OutDataTypeStr=Inherit: Same as first input
  Trigonometric Function : Trigonometry  Operator=cos
  adaptive filter : Subsystem
  adaptive mean : Subsystem
  alpha (rad) : Outport
  wt : Outport  Port=2
  wires:
  freq (pu)/1 -> Gain2/1
  Gain2/1 -> adaptive filter/2(freq (Hz)), adaptive mean/2(freq (Hz)), Gain/1
  Trigonometric Function/1 -> Product/2
  adaptive mean/1(y) -> alpha (rad)/1
  Integrator1/1 -> Gain1/1
  Gain1/1 -> Sum1/1, adaptive mean/1(u)
  Sum1/1 -> Trigonometric Function/1
  Integrator/1 -> Sum1/2, wt/1
  Gain/1 -> Integrator/1
  adaptive filter/1(y) -> Integrator1/1
  Product/1 -> adaptive filter/1(u)
  v (pu)/1 -> IC/1
  IC/1 -> Product/1

== system Feeder_1/SM_NG/Single-Phase Dynamic Load55/model/Positive Sequence  current ==
  note: I1= (S/V1)'
  V1(pu) : Inport
  S_ext : Inport  Port=2
  Conj1 : Math  Operator=conj  SaturateOnIntegerOverflow=on
  Product : Product  Inputs=/*  SaturateOnIntegerOverflow=on  InputSameDT=on  OutDataTypeStr=Inherit: Same as first input
  pu>V : Gain  Gain=Vnom/sqrt(2)  SaturateOnIntegerOverflow=on  OutDataTypeStr=Inherit: Same as input  ParamDataTypeStr=Inherit: Same as input
  I1(A) : Outport
  wires:
  V1(pu)/1 -> pu>V/1
  Product/1 -> Conj1/1
  Conj1/1 -> I1(A)/1
  S_ext/1 -> Product/2
  pu>V/1 -> Product/1

== system Feeder_1/SM_NG/Single-Phase Dynamic Load56/model/Break  Alg. Loop1 ==
  In : Inport
  Complex to Real-Imag : ComplexToRealImag
  Real-Imag to Complex : RealImagToComplex
  imag : simulink_extras/Additional Linear/Transfer Fcn (with initial outputs)  N=[1]  D="[100e-6  1]"  Y0=imag(I1_init*exp(-j*Pha_V0*pi/180))  U0=imag(I1_init*exp(-j*Pha_V0*pi/180))
  real : simulink_extras/Additional Linear/Transfer Fcn (with initial outputs)  N=[1]  D="[100e-6  1]"  Y0=real(I1_init*exp(-j*Pha_V0*pi/180))  U0=real(I1_init*exp(-j*Pha_V0*pi/180))
  Out : Outport
  wires:
  Complex to Real-Imag/2 -> imag/1
  Complex to Real-Imag/1 -> real/1
  Real-Imag to Complex/1 -> Out/1
  In/1 -> Complex to Real-Imag/1
  imag/1 -> Real-Imag to Complex/2
  real/1 -> Real-Imag to Complex/1

== system Feeder_1/SM_NG/Single-Phase Dynamic Load56/model/PLL ==
  v (pu) : Inport
  freq (pu) : Inport  Port=2
  Gain : Gain  Gain=2*pi
  Gain1 : Gain  Gain=500
  Gain2 : Gain  Gain=freq
  IC : InitialCondition
  Integrator : Integrator
  Integrator1 : Integrator
  Product : Product  Inputs=**  RndMeth=Zero
  Sum1 : Sum  SaturateOnIntegerOverflow=on  InputSameDT=on  OutDataTypeStr=Inherit: Same as first input
  Trigonometric Function : Trigonometry  Operator=cos
  adaptive filter : Subsystem
  adaptive mean : Subsystem
  alpha (rad) : Outport
  wt : Outport  Port=2
  wires:
  freq (pu)/1 -> Gain2/1
  Gain2/1 -> adaptive filter/2(freq (Hz)), adaptive mean/2(freq (Hz)), Gain/1
  Trigonometric Function/1 -> Product/2
  adaptive mean/1(y) -> alpha (rad)/1
  Integrator1/1 -> Gain1/1
  Gain1/1 -> Sum1/1, adaptive mean/1(u)
  Sum1/1 -> Trigonometric Function/1
  Integrator/1 -> Sum1/2, wt/1
  Gain/1 -> Integrator/1
  adaptive filter/1(y) -> Integrator1/1
  Product/1 -> adaptive filter/1(u)
  v (pu)/1 -> IC/1
  IC/1 -> Product/1

== system Feeder_1/SM_NG/Single-Phase Dynamic Load56/model/Positive Sequence  current ==
  note: I1= (S/V1)'
  V1(pu) : Inport
  S_ext : Inport  Port=2
  Conj1 : Math  Operator=conj  SaturateOnIntegerOverflow=on
  Product : Product  Inputs=/*  SaturateOnIntegerOverflow=on  InputSameDT=on  OutDataTypeStr=Inherit: Same as first input
  pu>V : Gain  Gain=Vnom/sqrt(2)  SaturateOnIntegerOverflow=on  OutDataTypeStr=Inherit: Same as input  ParamDataTypeStr=Inherit: Same as input
  I1(A) : Outport
  wires:
  V1(pu)/1 -> pu>V/1
  Product/1 -> Conj1/1
  Conj1/1 -> I1(A)/1
  S_ext/1 -> Product/2
  pu>V/1 -> Product/1

== system Feeder_1/SM_NG/Single-Phase Dynamic Load57/model/Break  Alg. Loop1 ==
  In : Inport
  Complex to Real-Imag : ComplexToRealImag
  Real-Imag to Complex : RealImagToComplex
  imag : simulink_extras/Additional Linear/Transfer Fcn (with initial outputs)  N=[1]  D="[100e-6  1]"  Y0=imag(I1_init*exp(-j*Pha_V0*pi/180))  U0=imag(I1_init*exp(-j*Pha_V0*pi/180))
  real : simulink_extras/Additional Linear/Transfer Fcn (with initial outputs)  N=[1]  D="[100e-6  1]"  Y0=real(I1_init*exp(-j*Pha_V0*pi/180))  U0=real(I1_init*exp(-j*Pha_V0*pi/180))
  Out : Outport
  wires:
  Complex to Real-Imag/2 -> imag/1
  Complex to Real-Imag/1 -> real/1
  Real-Imag to Complex/1 -> Out/1
  In/1 -> Complex to Real-Imag/1
  imag/1 -> Real-Imag to Complex/2
  real/1 -> Real-Imag to Complex/1

== system Feeder_1/SM_NG/Single-Phase Dynamic Load57/model/PLL ==
  v (pu) : Inport
  freq (pu) : Inport  Port=2
  Gain : Gain  Gain=2*pi
  Gain1 : Gain  Gain=500
  Gain2 : Gain  Gain=freq
  IC : InitialCondition
  Integrator : Integrator
  Integrator1 : Integrator
  Product : Product  Inputs=**  RndMeth=Zero
  Sum1 : Sum  SaturateOnIntegerOverflow=on  InputSameDT=on  OutDataTypeStr=Inherit: Same as first input
  Trigonometric Function : Trigonometry  Operator=cos
  adaptive filter : Subsystem
  adaptive mean : Subsystem
  alpha (rad) : Outport
  wt : Outport  Port=2
  wires:
  freq (pu)/1 -> Gain2/1
  Gain2/1 -> adaptive filter/2(freq (Hz)), adaptive mean/2(freq (Hz)), Gain/1
  Trigonometric Function/1 -> Product/2
  adaptive mean/1(y) -> alpha (rad)/1
  Integrator1/1 -> Gain1/1
  Gain1/1 -> Sum1/1, adaptive mean/1(u)
  Sum1/1 -> Trigonometric Function/1
  Integrator/1 -> Sum1/2, wt/1
  Gain/1 -> Integrator/1
  adaptive filter/1(y) -> Integrator1/1
  Product/1 -> adaptive filter/1(u)
  v (pu)/1 -> IC/1
  IC/1 -> Product/1

== system Feeder_1/SM_NG/Single-Phase Dynamic Load57/model/Positive Sequence  current ==
  note: I1= (S/V1)'
  V1(pu) : Inport
  S_ext : Inport  Port=2
  Conj1 : Math  Operator=conj  SaturateOnIntegerOverflow=on
  Product : Product  Inputs=/*  SaturateOnIntegerOverflow=on  InputSameDT=on  OutDataTypeStr=Inherit: Same as first input
  pu>V : Gain  Gain=Vnom/sqrt(2)  SaturateOnIntegerOverflow=on  OutDataTypeStr=Inherit: Same as input  ParamDataTypeStr=Inherit: Same as input
  I1(A) : Outport
  wires:
  V1(pu)/1 -> pu>V/1
  Product/1 -> Conj1/1
  Conj1/1 -> I1(A)/1
  S_ext/1 -> Product/2
  pu>V/1 -> Product/1

== system Feeder_1/SM_NG/Single-Phase Dynamic Load58/model/Break  Alg. Loop1 ==
  In : Inport
  Complex to Real-Imag : ComplexToRealImag
  Real-Imag to Complex : RealImagToComplex
  imag : simulink_extras/Additional Linear/Transfer Fcn (with initial outputs)  N=[1]  D="[100e-6  1]"  Y0=imag(I1_init*exp(-j*Pha_V0*pi/180))  U0=imag(I1_init*exp(-j*Pha_V0*pi/180))
  real : simulink_extras/Additional Linear/Transfer Fcn (with initial outputs)  N=[1]  D="[100e-6  1]"  Y0=real(I1_init*exp(-j*Pha_V0*pi/180))  U0=real(I1_init*exp(-j*Pha_V0*pi/180))
  Out : Outport
  wires:
  Complex to Real-Imag/2 -> imag/1
  Complex to Real-Imag/1 -> real/1
  Real-Imag to Complex/1 -> Out/1
  In/1 -> Complex to Real-Imag/1
  imag/1 -> Real-Imag to Complex/2
  real/1 -> Real-Imag to Complex/1

== system Feeder_1/SM_NG/Single-Phase Dynamic Load58/model/PLL ==
  v (pu) : Inport
  freq (pu) : Inport  Port=2
  Gain : Gain  Gain=2*pi
  Gain1 : Gain  Gain=500
  Gain2 : Gain  Gain=freq
  IC : InitialCondition
  Integrator : Integrator
  Integrator1 : Integrator
  Product : Product  Inputs=**  RndMeth=Zero
  Sum1 : Sum  SaturateOnIntegerOverflow=on  InputSameDT=on  OutDataTypeStr=Inherit: Same as first input
  Trigonometric Function : Trigonometry  Operator=cos
  adaptive filter : Subsystem
  adaptive mean : Subsystem
  alpha (rad) : Outport
  wt : Outport  Port=2
  wires:
  freq (pu)/1 -> Gain2/1
  Gain2/1 -> adaptive filter/2(freq (Hz)), adaptive mean/2(freq (Hz)), Gain/1
  Trigonometric Function/1 -> Product/2
  adaptive mean/1(y) -> alpha (rad)/1
  Integrator1/1 -> Gain1/1
  Gain1/1 -> Sum1/1, adaptive mean/1(u)
  Sum1/1 -> Trigonometric Function/1
  Integrator/1 -> Sum1/2, wt/1
  Gain/1 -> Integrator/1
  adaptive filter/1(y) -> Integrator1/1
  Product/1 -> adaptive filter/1(u)
  v (pu)/1 -> IC/1
  IC/1 -> Product/1

== system Feeder_1/SM_NG/Single-Phase Dynamic Load58/model/Positive Sequence  current ==
  note: I1= (S/V1)'
  V1(pu) : Inport
  S_ext : Inport  Port=2
  Conj1 : Math  Operator=conj  SaturateOnIntegerOverflow=on
  Product : Product  Inputs=/*  SaturateOnIntegerOverflow=on  InputSameDT=on  OutDataTypeStr=Inherit: Same as first input
  pu>V : Gain  Gain=Vnom/sqrt(2)  SaturateOnIntegerOverflow=on  OutDataTypeStr=Inherit: Same as input  ParamDataTypeStr=Inherit: Same as input
  I1(A) : Outport
  wires:
  V1(pu)/1 -> pu>V/1
  Product/1 -> Conj1/1
  Conj1/1 -> I1(A)/1
  S_ext/1 -> Product/2
  pu>V/1 -> Product/1

== system Feeder_1/SM_NG/Single-Phase Dynamic Load59/model/Break  Alg. Loop1 ==
  In : Inport
  Complex to Real-Imag : ComplexToRealImag
  Real-Imag to Complex : RealImagToComplex
  imag : simulink_extras/Additional Linear/Transfer Fcn (with initial outputs)  N=[1]  D="[100e-6  1]"  Y0=imag(I1_init*exp(-j*Pha_V0*pi/180))  U0=imag(I1_init*exp(-j*Pha_V0*pi/180))
  real : simulink_extras/Additional Linear/Transfer Fcn (with initial outputs)  N=[1]  D="[100e-6  1]"  Y0=real(I1_init*exp(-j*Pha_V0*pi/180))  U0=real(I1_init*exp(-j*Pha_V0*pi/180))
  Out : Outport
  wires:
  Complex to Real-Imag/2 -> imag/1
  Complex to Real-Imag/1 -> real/1
  Real-Imag to Complex/1 -> Out/1
  In/1 -> Complex to Real-Imag/1
  imag/1 -> Real-Imag to Complex/2
  real/1 -> Real-Imag to Complex/1

== system Feeder_1/SM_NG/Single-Phase Dynamic Load59/model/PLL ==
  v (pu) : Inport
  freq (pu) : Inport  Port=2
  Gain : Gain  Gain=2*pi
  Gain1 : Gain  Gain=500
  Gain2 : Gain  Gain=freq
  IC : InitialCondition
  Integrator : Integrator
  Integrator1 : Integrator
  Product : Product  Inputs=**  RndMeth=Zero
  Sum1 : Sum  SaturateOnIntegerOverflow=on  InputSameDT=on  OutDataTypeStr=Inherit: Same as first input
  Trigonometric Function : Trigonometry  Operator=cos
  adaptive filter : Subsystem
  adaptive mean : Subsystem
  alpha (rad) : Outport
  wt : Outport  Port=2
  wires:
  freq (pu)/1 -> Gain2/1
  Gain2/1 -> adaptive filter/2(freq (Hz)), adaptive mean/2(freq (Hz)), Gain/1
  Trigonometric Function/1 -> Product/2
  adaptive mean/1(y) -> alpha (rad)/1
  Integrator1/1 -> Gain1/1
  Gain1/1 -> Sum1/1, adaptive mean/1(u)
  Sum1/1 -> Trigonometric Function/1
  Integrator/1 -> Sum1/2, wt/1
  Gain/1 -> Integrator/1
  adaptive filter/1(y) -> Integrator1/1
  Product/1 -> adaptive filter/1(u)
  v (pu)/1 -> IC/1
  IC/1 -> Product/1

== system Feeder_1/SM_NG/Single-Phase Dynamic Load59/model/Positive Sequence  current ==
  note: I1= (S/V1)'
  V1(pu) : Inport
  S_ext : Inport  Port=2
  Conj1 : Math  Operator=conj  SaturateOnIntegerOverflow=on
  Product : Product  Inputs=/*  SaturateOnIntegerOverflow=on  InputSameDT=on  OutDataTypeStr=Inherit: Same as first input
  pu>V : Gain  Gain=Vnom/sqrt(2)  SaturateOnIntegerOverflow=on  OutDataTypeStr=Inherit: Same as input  ParamDataTypeStr=Inherit: Same as input
  I1(A) : Outport
  wires:
  V1(pu)/1 -> pu>V/1
  Product/1 -> Conj1/1
  Conj1/1 -> I1(A)/1
  S_ext/1 -> Product/2
  pu>V/1 -> Product/1

== system Feeder_1/SM_NG/Single-Phase Dynamic Load60/model/Break  Alg. Loop1 ==
  In : Inport
  Complex to Real-Imag : ComplexToRealImag
  Real-Imag to Complex : RealImagToComplex
  imag : simulink_extras/Additional Linear/Transfer Fcn (with initial outputs)  N=[1]  D="[100e-6  1]"  Y0=imag(I1_init*exp(-j*Pha_V0*pi/180))  U0=imag(I1_init*exp(-j*Pha_V0*pi/180))
  real : simulink_extras/Additional Linear/Transfer Fcn (with initial outputs)  N=[1]  D="[100e-6  1]"  Y0=real(I1_init*exp(-j*Pha_V0*pi/180))  U0=real(I1_init*exp(-j*Pha_V0*pi/180))
  Out : Outport
  wires:
  Complex to Real-Imag/2 -> imag/1
  Complex to Real-Imag/1 -> real/1
  Real-Imag to Complex/1 -> Out/1
  In/1 -> Complex to Real-Imag/1
  imag/1 -> Real-Imag to Complex/2
  real/1 -> Real-Imag to Complex/1

== system Feeder_1/SM_NG/Single-Phase Dynamic Load60/model/PLL ==
  v (pu) : Inport
  freq (pu) : Inport  Port=2
  Gain : Gain  Gain=2*pi
  Gain1 : Gain  Gain=500
  Gain2 : Gain  Gain=freq
  IC : InitialCondition
  Integrator : Integrator
  Integrator1 : Integrator
  Product : Product  Inputs=**  RndMeth=Zero
  Sum1 : Sum  SaturateOnIntegerOverflow=on  InputSameDT=on  OutDataTypeStr=Inherit: Same as first input
  Trigonometric Function : Trigonometry  Operator=cos
  adaptive filter : Subsystem
  adaptive mean : Subsystem
  alpha (rad) : Outport
  wt : Outport  Port=2
  wires:
  freq (pu)/1 -> Gain2/1
  Gain2/1 -> adaptive filter/2(freq (Hz)), adaptive mean/2(freq (Hz)), Gain/1
  Trigonometric Function/1 -> Product/2
  adaptive mean/1(y) -> alpha (rad)/1
  Integrator1/1 -> Gain1/1
  Gain1/1 -> Sum1/1, adaptive mean/1(u)
  Sum1/1 -> Trigonometric Function/1
  Integrator/1 -> Sum1/2, wt/1
  Gain/1 -> Integrator/1
  adaptive filter/1(y) -> Integrator1/1
  Product/1 -> adaptive filter/1(u)
  v (pu)/1 -> IC/1
  IC/1 -> Product/1

== system Feeder_1/SM_NG/Single-Phase Dynamic Load60/model/Positive Sequence  current ==
  note: I1= (S/V1)'
  V1(pu) : Inport
  S_ext : Inport  Port=2
  Conj1 : Math  Operator=conj  SaturateOnIntegerOverflow=on
  Product : Product  Inputs=/*  SaturateOnIntegerOverflow=on  InputSameDT=on  OutDataTypeStr=Inherit: Same as first input
  pu>V : Gain  Gain=Vnom/sqrt(2)  SaturateOnIntegerOverflow=on  OutDataTypeStr=Inherit: Same as input  ParamDataTypeStr=Inherit: Same as input
  I1(A) : Outport
  wires:
  V1(pu)/1 -> pu>V/1
  Product/1 -> Conj1/1
  Conj1/1 -> I1(A)/1
  S_ext/1 -> Product/2
  pu>V/1 -> Product/1
